simulink model "tp2_3"  (R2023b)
settings: Solver=VariableStepAuto  StartTime=0.0  StopTime=50.0  RelTol=1e-3
settings Model: Creator=rusha  LastModifiedBy=rusha

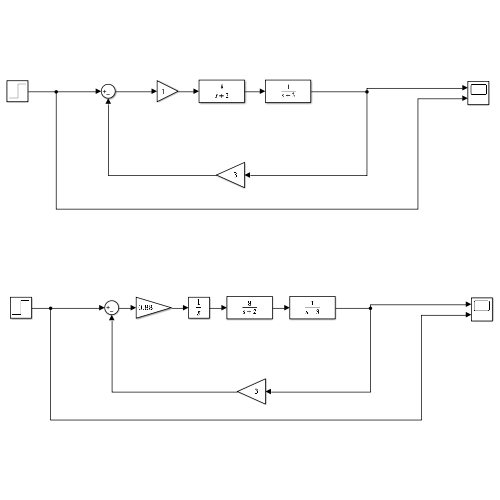
[thumbnail: Simulink's stored preview of the top-level diagram]
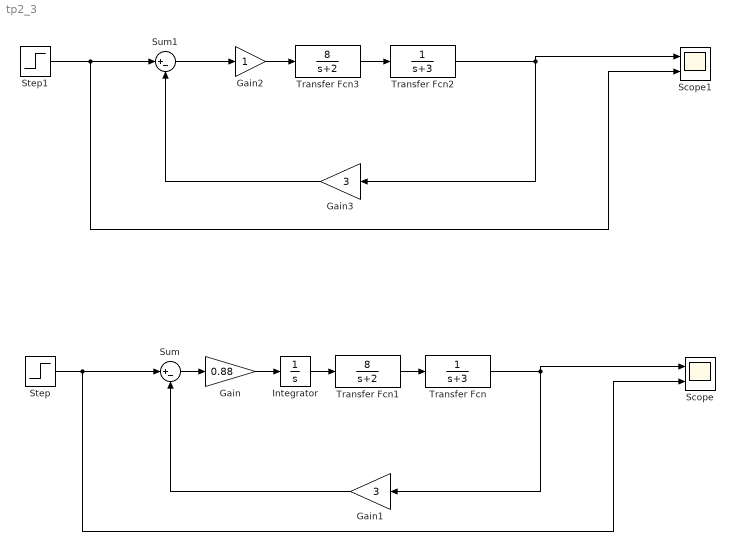
== system tp2_3 ==
  Gain : Gain  Gain=0.88
  Gain1 : Gain  Gain=3
  Gain2 : Gain
  Gain3 : Gain  Gain=3
  Integrator : Integrator
  Scope : Scope  NumInputPorts=2
  Scope1 : Scope  NumInputPorts=2
  Step : Step  SampleTime=0
  Step1 : Step  SampleTime=0
  Sum : Sum  Inputs=|+-
  Sum1 : Sum  Inputs=|+-
  Transfer Fcn : TransferFcn  Denominator=[1 3]
  Transfer Fcn1 : TransferFcn  Numerator=[8]  Denominator=[1 2]
  Transfer Fcn2 : TransferFcn  Denominator=[1 3]
  Transfer Fcn3 : TransferFcn  Numerator=[8]  Denominator=[1 2]
  wires:
  Transfer Fcn/1 -> Gain1/1, Scope/1
  Gain1/1 -> Sum/2
  Step/1 -> Scope/2, Sum/1
  Integrator/1 -> Transfer Fcn1/1
  Transfer Fcn1/1 -> Transfer Fcn/1
  Gain/1 -> Integrator/1
  Sum/1 -> Gain/1
  Step1/1 -> Scope1/2, Sum1/1
  Sum1/1 -> Gain2/1
  Transfer Fcn3/1 -> Transfer Fcn2/1
  Gain3/1 -> Sum1/2
  Transfer Fcn2/1 -> Gain3/1, Scope1/1
  Gain2/1 -> Transfer Fcn3/1
